simulink model "sldemo_enginewc"  (R2021a)
settings: Solver=ode23s  StartTime=0.0  StopTime=10  RelTol=1e-3  AbsTol=1e-6
PreLoadFcn:
  | Kp =0.0614; Ki = 0.0723;
libraries: pid_lib x1
Description:
  | Engine Timing Model With Closed Loop Control
  | 
  | This example shows how to use triggered subsystems in Simulink(R) to model
  | engine timing, including a feedback controller. Different subsystems in the diagram
  | model the mathematical representation of various automotive systems, including
  | the following:
  | 
  | * Throttle and manifold
  | * Compression
  | * Combustion
  | * Vehicle dynamics
  | * Valve timing
  | * Controller
  | 
  | The valve timing subsystem generates a signal that triggers the Controller and
  | Compression subsystems twice per revolution of the crank (calculated from the
  | crank speed.) A speed set point (in rpm) from the Step block drives the simulation.
  | The controller calculates the necessary throttle angle based on the desired rpm
  | and the crank speed that is calculated by the vehicle dynamics. After you run
  | the simulation, the Scopes show the engine speed and the throttle angle
  | compared to the load torque.
settings Model: ExtModeTrigMode=oneshot  ExtModeArmWhenConnect=off  ExtModeAutoUpdateStatusClock=off  Creator=The MathWorks, Inc.  LastModifiedBy=The MathWorks, Inc.
settings SolverCC: AutoScaleAbsTol=off  AlgebraicLoopSolver=TrustRegion
settings DataIOCC: ExternalInput=[]  InitialState=[]  SaveFormat=Array  SaveOutput=off  SaveTime=off  ReturnWorkspaceOutputs=off  StateSaveName=x  TimeSaveName=t  OutputSaveName=y  SignalLoggingName=sldemo_enginewc_output
settings OptimizationCC: BlockReduction=off  ExpressionDepthLimit=2147483647  InitFltsAndDblsToZero=on  LifeSpan=inf  BufferReusableBoundary=off
settings DebuggingCC: SaveWithParameterizedLinksMsg=none  UnderspecifiedInitializationDetection=Classic  MergeDetectMultiDrivingBlocksExec=none  SignalResolutionControl=TryResolveAllWithWarning  MultiTaskDSMMsg=warning  MultiTaskCondExecSysMsg=none  SigSpecEnsureSampleTimeMsg=none  IntegerOverflowMsg=none  FcnCallInpInsideContextMsg=warning  BusObjectLabelMismatch=none  AllowSymbolicDim=off  StateNameClashWarn=warning  SFUnexpectedBacktrackingDiag=warning  SFNoUnconditionalDefaultTransitionDiag=warning  SFExecutionAtInitializationDiag=none  SFMachineParentedDataDiag=warning  IntegerSaturationMsg=none  ArithmeticOperatorsInVariantConditions=warning
settings HardwareCC: ProdBitPerPointer=32  ProdBitPerSizeT=32  ProdBitPerPtrDiffT=32  ProdLargestAtomicFloat=None  ProdIntDivRoundTo=Undefined  ProdEndianess=Unspecified  ProdWordSize=32  ProdHWDeviceType=32-bit Generic
settings ModelReferenceCC: PropagateSignalLabelsOutOfModel=off
settings SFSimCC: SimUseLocalCustomCode=off  CustomCodeUndefinedFunction=UseInterfaceOnly
settings RTWCC: Description=Generic Real-Time Target  RTWUseLocalCustomCode=off
settings CodeAppCC: StateflowObjectComments=on
settings GRTTargetCC: TargetFcnLib=ansi_tfl_tmw.mat  TargetLangStandard=C89/C90 (ANSI)  CombineOutputUpdateFcns=off  GRTInterface=on
settings ConfigComp: CovMetricSettings=d  CovSaveCumulativeToWorkspaceVar=on  CovSaveSingleToWorkspaceVar=on  CovExternalEMLEnable=off

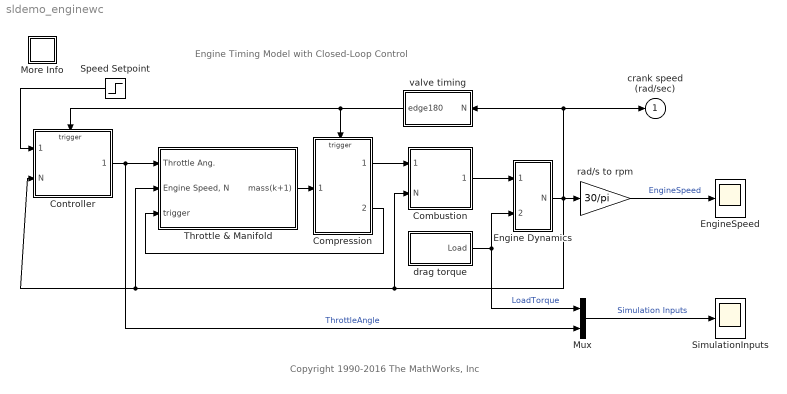
== system sldemo_enginewc ==
  note: Engine Timing Model with Closed-Loop Control
  note: Copyright 1990-2016 The MathWorks, Inc
  Combustion : Subsystem
  Compression : Subsystem  TreatAsAtomicUnit=on
  Controller : Subsystem  TreatAsAtomicUnit=on
  Engine Dynamics : Subsystem
  EngineSpeed : Scope
  More Info : Subsystem
      settings: OpenFcn=showExample('simulink_automotive/EngineTimingModelWithClosedLoopControlExample')
      mask Display: disp('?')
  Mux : Mux  Inputs=2
  SimulationInputs : Scope
  Speed Setpoint : Step  Time=5  Before=2000  After=3000  SampleTime=0
  Throttle & Manifold : Subsystem
  drag torque : Subsystem
  rad/s to rpm : Gain  Gain=30/pi  SaturateOnIntegerOverflow=on  OutDataTypeStr=Inherit: Same as input  ParamDataTypeStr=Inherit: Same as input
  valve timing : Subsystem
  crank speed (rad/sec) : Outport  InitialOutput=0
  wires:
  Speed Setpoint/1 -> Controller/1(Desired rpm)
  drag torque/1(Load) -> Mux/1, Engine Dynamics/2(Tload)  "LoadTorque"
  Controller/1(Throttle Ang.) -> Mux/2, Throttle & Manifold/1(Throttle Ang.)  "ThrottleAngle"
  Compression/1(mass(k)) -> Combustion/1(Air Charge)
  valve timing/1(edge180) -> Controller/Trigger, Compression/Trigger
  Combustion/1(Torque) -> Engine Dynamics/1(Teng)
  Engine Dynamics/1(N) -> rad/s to rpm/1, crank speed (rad/sec)/1, valve timing/1(N), Controller/2(N), Throttle & Manifold/2("Engine Speed, N"), Combustion/2(N)
  rad/s to rpm/1 -> EngineSpeed/1  "EngineSpeed"
  Mux/1 -> SimulationInputs/1  "Simulation Inputs"
  Throttle & Manifold/1(mass(k+1)) -> Compression/1(mass(k+1))
  Compression/2(trigger) -> Throttle & Manifold/3(trigger)

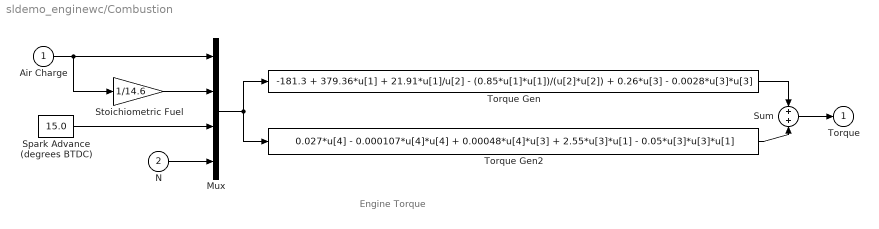
== system sldemo_enginewc/Combustion ==
  note: Engine Torque
  Air Charge : Inport
  N : Inport  Port=2
  Mux : Mux
  Spark Advance (degrees BTDC) : Constant  Value=15.0
  Stoichiometric Fuel : Gain  Gain=1/14.6  SaturateOnIntegerOverflow=on  OutDataTypeStr=Inherit: Same as input  ParamDataTypeStr=Inherit: Same as input
  Sum : Sum  InputSameDT=on  SaturateOnIntegerOverflow=on  OutDataTypeStr=Inherit: Same as first input
  Torque Gen : Fcn  Expr=-181.3 + 379.36*u[1] + 21.91*u[1]/u[2] - (0.85*u[1]*u[1])/(u[2]*u[2]) + 0.26*u[3] - 0.0028*u[3]*u[3]
  Torque Gen2 : Fcn  Expr=0.027*u[4] - 0.000107*u[4]*u[4] + 0.00048*u[4]*u[3] + 2.55*u[3]*u[1] - 0.05*u[3]*u[3]*u[1]
  Torque : Outport  InitialOutput=0
  wires:
  Stoichiometric Fuel/1 -> Mux/2
  Spark Advance (degrees BTDC)/1 -> Mux/3
  N/1 -> Mux/4
  Air Charge/1 -> Stoichiometric Fuel/1, Mux/1
  Mux/1 -> Torque Gen/1, Torque Gen2/1
  Torque Gen2/1 -> Sum/2
  Torque Gen/1 -> Sum/1
  Sum/1 -> Torque/1

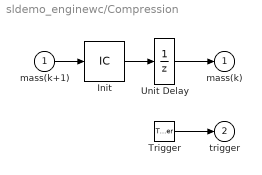
== system sldemo_enginewc/Compression ==
  mass(k+1) : Inport
  Trigger : TriggerPort  TriggerType=either  VariantControl=Variant  ShowOutputPort=on
  Init : InitialCondition  Value=0.152
  Unit Delay : UnitDelay  InitialCondition=0.152  SampleTime=-1  HasFrameUpgradeWarning=on
  mass(k) : Outport  InitialOutput=0.152
  trigger : Outport  Port=2  InitialOutput=-1
  wires:
  Init/1 -> Unit Delay/1
  mass(k+1)/1 -> Init/1
  Unit Delay/1 -> mass(k)/1
  Trigger/1 -> trigger/1

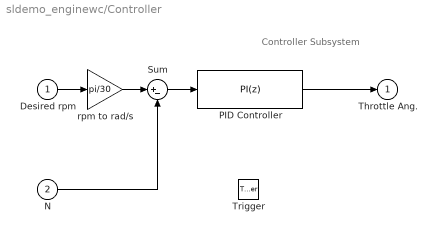
== system sldemo_enginewc/Controller ==
  note: Controller Subsystem
  Desired rpm : Inport
  N : Inport  Port=2
  Trigger : TriggerPort  TriggerType=either  VariantControl=Variant
  PID Controller : pid_lib/PID Controller  Controller=PI  Form=Parallel  TimeDomain=Discrete-time  UseExternalTs=off  SampleTime=-1  IntegratorMethod=Forward Euler  FilterMethod=Forward Euler  ControllerParametersSource=internal  P=Kp  I=Ki  D=0  UseFilter=on  N=100  TunerSelectOption=Transfer Function Based (PID Tuner App)  InitialConditionSource=internal  InitialConditionForIntegrator=8.973  InitialConditionForFilter=0  DifferentiatorICPrevScaledInput=0  ExternalReset=none  TrackingMode=off  Kt=1  LimitOutput=on  SatLimitsSource=internal  UpperSaturationLimit=70  LowerSaturationLimit=0  LinearizeAsGain=on  AntiWindupMode=clamping  Kb=1  POutMin=[]  POutMax=[]  IOutMin=[]  IOutMax=[]  DOutMin=[]  DOutMax=[]  NOutMin=[]  NOutMax=[]  SumOutMin=[]  SumOutMax=[]  SaturationOutMin=[]  SaturationOutMax=[]  PParamMin=[]  PParamMax=[]  IParamMin=[]  IParamMax=[]  DParamMin=[]  DParamMax=[]  NParamMin=[]  NParamMax=[]  KbParamMin=[]  KbParamMax=[]  KtParamMin=[]  KtParamMax=[]  KbOutMin=[]  KbOutMax=[]  KtOutMin=[]  KtOutMax=[]  IntegratorOutMin=[]  IntegratorOutMax=[]  FilterOutMin=[]  FilterOutMax=[]  SumI1OutMin=[]  SumI1OutMax=[]  SumI2OutMin=[]  SumI2OutMax=[]  SumI3OutMin=[]  SumI3OutMax=[]  SumI4OutMin=[]  SumI4OutMax=[]  SumDOutMin=[]  SumDOutMax=[]  DifferentiatorOutMin=[]  DifferentiatorOutMax=[]  FilterDiffOutCoefMin=[]  FilterDiffOutCoefMax=[]  ReciprocalOutMin=[]  ReciprocalOutMax=[]  SumDenOutMin=[]  SumDenOutMax=[]  SumNumOutMin=[]  SumNumOutMax=[]  DivideOutMin=[]  DivideOutMax=[]  UdiffTsProdOutMin=[]  UdiffTsProdOutMax=[]  NTsProdOutMin=[]  NTsProdOutMax=[]  UintegralTsProdOutMin=[]  UintegralTsProdOutMax=[]  UngainTsProdOutMin=[]  UngainTsProdOutMax=[]  IntegratorContinuousStateAttributes=''  IntegratorStateMustResolveToSignalObject=off  IntegratorRTWStateStorageClass=Auto  FilterContinuousStateAttributes=''  FilterStateMustResolveToSignalObject=off  FilterRTWStateStorageClass=Auto  ParallelPVariant=InternalParameters  IdealPVariant=Disabled  IVariant=InternalParameters  DVariant=Disabled  IntegratorVariant=Discrete  SatVariant=Enabled  AWVariant=DiscClampingParallel  PCopyVariant=Disabled  TRVariant=Disabled  FdbkBlocksVariant=Forward  IdealPFdbkVariant=Disabled  SatFdbkVariant=Disabled  DerivativeFilterVariant=Disabled  NVariant=Disabled  NCopyVariant=Disabled_SignalSpec  FilterICVariant=Disabled  IntegratorICVariant=InternalICs  ExternalResetVariant=Disabled  TRSumVariant=Passthrough  SumFdbkVariant=Disabled  SumVariant=Sum_PI  TsampFilterVariant=InternalTs  TsampNgainVariant=Passthrough  TsampIntegralVariant=Passthrough  ExternalSaturationOutDataTypeStr=Inherit: Same as second input
  Sum : Sum  Inputs=|+-  InputSameDT=on  SaturateOnIntegerOverflow=on  OutDataTypeStr=Inherit: Same as first input
  rpm to rad/s : Gain  Gain=pi/30  SaturateOnIntegerOverflow=on  OutDataTypeStr=Inherit: Same as input  ParamDataTypeStr=Inherit: Same as input
  Throttle Ang. : Outport  InitialOutput=8.973
  wires:
  rpm to rad/s/1 -> Sum/1
  N/1 -> Sum/2
  Desired rpm/1 -> rpm to rad/s/1
  Sum/1 -> PID Controller/1
  PID Controller/1 -> Throttle Ang./1

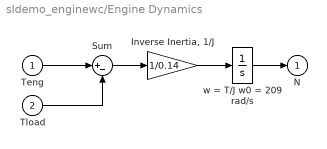
== system sldemo_enginewc/Engine Dynamics ==
  Teng : Inport
  Tload : Inport  Port=2
  "Inverse Inertia, 1/J" : Gain  Gain=1/0.14  SaturateOnIntegerOverflow=on  OutDataTypeStr=Inherit: Same as input  ParamDataTypeStr=Inherit: Same as input
  Sum : Sum  Inputs=|+-  InputSameDT=on  SaturateOnIntegerOverflow=on  OutDataTypeStr=Inherit: Same as first input
  w = T/J w0 = 209 rad/s : Integrator  InitialCondition=209.48
  N : Outport  InitialOutput=0
  wires:
  "Inverse Inertia, 1/J"/1 -> w = T/J w0 = 209 rad/s/1
  w = T/J w0 = 209 rad/s/1 -> N/1
  Sum/1 -> "Inverse Inertia, 1/J"/1
  Teng/1 -> Sum/1
  Tload/1 -> Sum/2

== system sldemo_enginewc/More Info ==

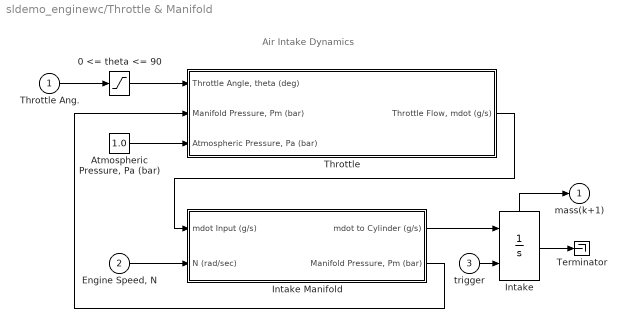
== system sldemo_enginewc/Throttle & Manifold ==
  note: Air Intake Dynamics
  Throttle Ang. : Inport
  "Engine Speed, N" : Inport  Port=2
  trigger : Inport  Port=3
  0 <= theta <= 90 : Saturate  UpperLimit=90  LowerLimit=0
  "Atmospheric Pressure, Pa (bar)" : Constant  Value=1.0
  Intake : Integrator  ExternalReset=either  ShowStatePort=on
  Intake Manifold : Subsystem
  Terminator : Terminator
  Throttle : Subsystem
  mass(k+1) : Outport  InitialOutput=0
  wires:
  0 <= theta <= 90/1 -> Throttle/1("Throttle Angle, theta (deg)")
  Throttle Ang./1 -> 0 <= theta <= 90/1
  Throttle/1("Throttle Flow, mdot (g/s)") -> Intake Manifold/1(mdot Input (g/s))
  "Engine Speed, N"/1 -> Intake Manifold/2(N (rad/sec))
  Intake Manifold/2("Manifold Pressure, Pm (bar)") -> Throttle/2("Manifold Pressure, Pm (bar)")
  Intake Manifold/1(mdot to Cylinder (g/s)) -> Intake/1
  "Atmospheric Pressure, Pa (bar)"/1 -> Throttle/3("Atmospheric Pressure, Pa (bar) ")
  Intake/State -> mass(k+1)/1
  trigger/1 -> Intake/2
  Intake/1 -> Terminator/1

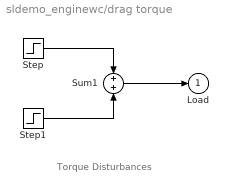
== system sldemo_enginewc/drag torque ==
  note: Torque Disturbances
  Step : Step  Time=2  Before=25  After=20  SampleTime=0
  Step1 : Step  Time=8  After=5  SampleTime=0
  Sum1 : Sum  InputSameDT=on  SaturateOnIntegerOverflow=on  OutDataTypeStr=Inherit: Same as first input
  Load : Outport  InitialOutput=0
  wires:
  Sum1/1 -> Load/1
  Step/1 -> Sum1/1
  Step1/1 -> Sum1/2

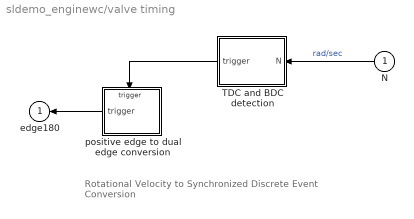
== system sldemo_enginewc/valve timing ==
  note: Rotational Velocity to Synchronized
      | Discrete Event Conversion
  N : Inport
  TDC and BDC detection : Subsystem
  positive edge to dual edge conversion : Subsystem  TreatAsAtomicUnit=on
  edge180 : Outport  InitialOutput=-1
  wires:
  TDC and BDC detection/1(trigger) -> positive edge to dual edge conversion/Trigger
  positive edge to dual edge conversion/1(trigger) -> edge180/1
  N/1 -> TDC and BDC detection/1(N)  "rad/sec"

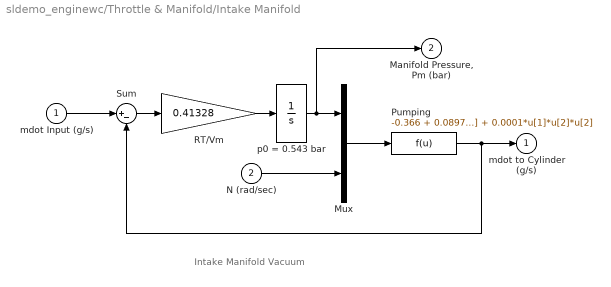
== system sldemo_enginewc/Throttle & Manifold/Intake Manifold ==
  note: Intake Manifold Vacuum
  mdot Input (g/s) : Inport
  N (rad/sec) : Inport  Port=2
  Mux : Mux  Inputs=2
  Pumping : Fcn  Expr=-0.366 + 0.08979*u[1]*u[2] - 0.0337*u[2]*u[1]*u[1] + 0.0001*u[1]*u[2]*u[2]
  RT/Vm : Gain  Gain=0.41328  SaturateOnIntegerOverflow=on  OutDataTypeStr=Inherit: Same as input  ParamDataTypeStr=Inherit: Same as input
  Sum : Sum  Inputs=|+-  InputSameDT=on  SaturateOnIntegerOverflow=on  OutDataTypeStr=Inherit: Same as first input
  p0 = 0.543 bar : Integrator  InitialCondition=.543
  mdot to Cylinder (g/s) : Outport  InitialOutput=0
  "Manifold Pressure, Pm (bar)" : Outport  Port=2  InitialOutput=0
  wires:
  mdot Input (g/s)/1 -> Sum/1
  RT/Vm/1 -> p0 = 0.543 bar/1
  N (rad/sec)/1 -> Mux/2
  Mux/1 -> Pumping/1
  p0 = 0.543 bar/1 -> Mux/1, "Manifold Pressure, Pm (bar)"/1
  Sum/1 -> RT/Vm/1
  Pumping/1 -> Sum/2, mdot to Cylinder (g/s)/1

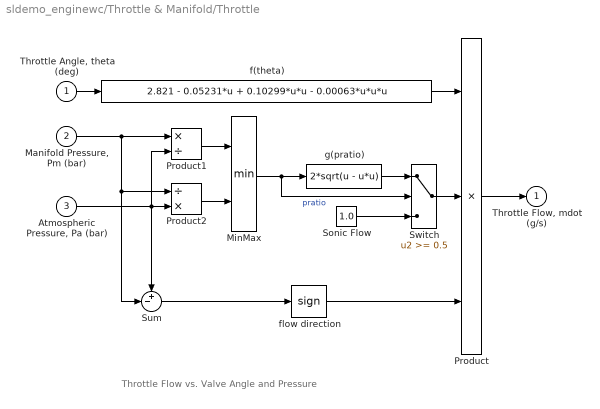
== system sldemo_enginewc/Throttle & Manifold/Throttle ==
  note: Throttle Flow vs. Valve Angle and Pressure
  "Throttle Angle, theta (deg)" : Inport
  "Manifold Pressure, Pm (bar)" : Inport  Port=2
  "Atmospheric Pressure, Pa (bar) " : Inport  Port=3
  MinMax : MinMax  Inputs=2  InputSameDT=on  SaturateOnIntegerOverflow=on
  Product : Product  Inputs=3  InputSameDT=on  RndMeth=Zero  SaturateOnIntegerOverflow=on  OutDataTypeStr=Inherit: Same as first input
  Product1 : Product  Inputs=*/  InputSameDT=on  RndMeth=Zero  SaturateOnIntegerOverflow=on  OutDataTypeStr=Inherit: Same as first input
  Product2 : Product  Inputs=/*  InputSameDT=on  RndMeth=Zero  SaturateOnIntegerOverflow=on  OutDataTypeStr=Inherit: Same as first input
  "Sonic Flow " : Constant  Value=1.0
  Sum : Sum  Inputs=+-|  InputSameDT=on  SaturateOnIntegerOverflow=on  OutDataTypeStr=Inherit: Same as first input
  Switch : Switch  Threshold=0.5  SaturateOnIntegerOverflow=on  InputSameDT=on
  f(theta) : Fcn  Expr=2.821 - 0.05231*u + 0.10299*u*u - 0.00063*u*u*u
  flow direction : Signum
  g(pratio) : Fcn  Expr=2*sqrt(u - u*u)
  "Throttle Flow, mdot (g/s)" : Outport  InitialOutput=0
  wires:
  "Manifold Pressure, Pm (bar)"/1 -> Sum/2, Product2/1, Product1/1
  Product2/1 -> MinMax/2
  Product1/1 -> MinMax/1
  "Atmospheric Pressure, Pa (bar) "/1 -> Sum/1, Product2/2, Product1/2
  g(pratio)/1 -> Switch/1
  "Sonic Flow "/1 -> Switch/3
  Switch/1 -> Product/2
  flow direction/1 -> Product/3
  Sum/1 -> flow direction/1
  MinMax/1 -> Switch/2, g(pratio)/1  "pratio"
  "Throttle Angle, theta (deg)"/1 -> f(theta)/1
  Product/1 -> "Throttle Flow, mdot (g/s)"/1
  f(theta)/1 -> Product/1

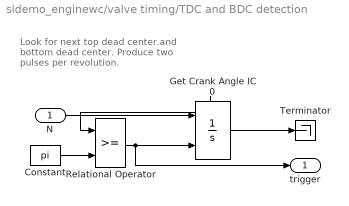
== system sldemo_enginewc/valve timing/TDC and BDC detection ==
  note: Look for next top dead center.and
      | bottom dead center.
      | Produce two pulses per revolution.
  N : Inport
  Constant : Constant  Value=pi
  Get Crank Angle IC 0 : Integrator  ExternalReset=rising  ShowStatePort=on
  Relational Operator : RelationalOperator  OutDataTypeStr=boolean  RndMeth=Nearest  InputSameDT=on
  Terminator : Terminator
  trigger : Outport  InitialOutput=0
  wires:
  N/1 -> Get Crank Angle IC 0/1
  Relational Operator/1 -> trigger/1, Get Crank Angle IC 0/2
  Constant/1 -> Relational Operator/2
  Get Crank Angle IC 0/State -> Relational Operator/1
  Get Crank Angle IC 0/1 -> Terminator/1

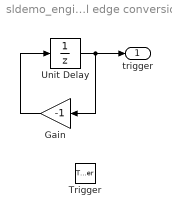
== system sldemo_enginewc/valve timing/positive edge to dual edge conversion ==
  Trigger : TriggerPort  VariantControl=Variant
  Gain : Gain  Gain=-1  SaturateOnIntegerOverflow=on  OutDataTypeStr=Inherit: Same as input  ParamDataTypeStr=Inherit: Same as input
  Unit Delay : UnitDelay  InitialCondition=1  SampleTime=-1  HasFrameUpgradeWarning=on
  trigger : Outport  InitialOutput=-1
  wires:
  Gain/1 -> Unit Delay/1
  Unit Delay/1 -> trigger/1, Gain/1
